simulink library "components"  (R2016a)
settings: Solver=VariableStepAuto  StartTime=0.0  StopTime=10.0  RelTol=1e-3
settings Model: Creator=noah.huesser  LastModifiedBy=noah.huesser
settings GRTTargetCC: GeneratePreprocessorConditionals=Use local settings

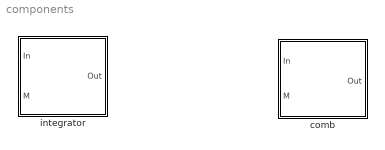
== system components ==
  comb : Subsystem
  integrator : Subsystem

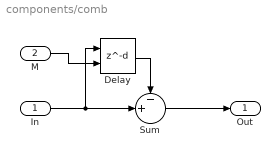
== system components/comb ==
  In : Inport
  M : Inport  Port=2
  Delay : Delay  DelayLengthSource=Input port  DelayLength=1  InitialCondition=0
      settings: InputPortMap=u0,p1
  Sum : Sum  Inputs=-+|
  Out : Outport
  wires:
  Sum/1 -> Out/1
  In/1 -> Sum/2, Delay/1
  Delay/1 -> Sum/1
  M/1 -> Delay/2

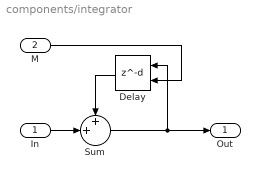
== system components/integrator ==
  In : Inport
  M : Inport  Port=2
  Delay : Delay  DelayLengthSource=Input port  DelayLength=1
      settings: InputPortMap=u0,p1
  Sum : Sum  Inputs=++|
  Out : Outport
  wires:
  In/1 -> Sum/2
  Delay/1 -> Sum/1
  Sum/1 -> Out/1, Delay/1
  M/1 -> Delay/2
